simulink model "hw32a"  (R2017a)
settings: Solver=VariableStepAuto  StartTime=0.0  StopTime=10.0  RelTol=1e-3
undefined symbols (not defined in the file): sigbuilder_block
settings Model: Creator=Soutrik  LastModifiedBy=Soutrik

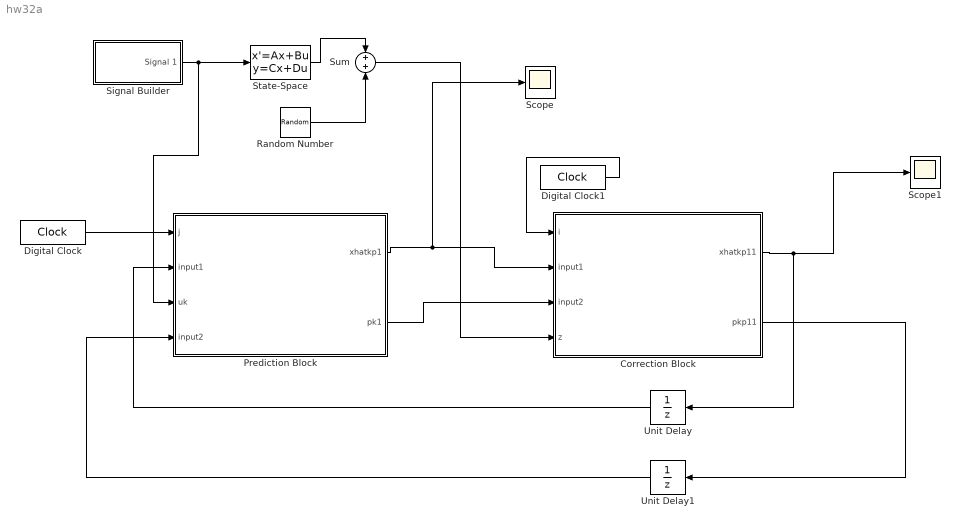
== system hw32a ==
  Correction Block : MATLAB Function  TreatAsAtomicUnit=on
  Digital Clock : DigitalClock  SampleTime=0.01
  Digital Clock1 : DigitalClock  SampleTime=0.01
  Prediction Block : MATLAB Function  TreatAsAtomicUnit=on
  Random Number : RandomNumber  Variance=[0.0001, 0.0000001, 0.00002, 0.00002]  SampleTime=0.01
  Scope : Scope
  Scope1 : Scope
  Signal Builder : Subsystem  Tag=STV Subsys  LoadFcn=sigbuilder_block('load');  StartFcn=sigbuilder_block('start');  StopFcn=sigbuilder_block('stop');  ClipboardFcn=sigbuilder_block('clipboard');  mask(Sigbuilder block){tuvar=[0:10]}
      mask help: Simulink:masks:SigbuilderBlock_MD
      mask init:
      | if ~strcmp(get_param(bdroot(gcbh),'SimulationStatus'),'stopped') tuvar = sigbuilder_block('maskInit'); end
      settings: CopyFcn=sigbuilder_block('copy');  DeleteFcn=sigbuilder_block('delete');  ModelCloseFcn=sigbuilder_block('modelClose');  PreSaveFcn=sigbuilder_block('preSave');  PauseFcn=sigbuilder_block('pause');  ContinueFcn=sigbuilder_block('continue');  NameChangeFcn=sigbuilder_block('namechange');  OpenFcn=sigbuilder_block('open',[300 184.875 550.5 400.125 ]);  CloseFcn=sigbuilder_block('close');
      mask Display: plot(0, 0, 100, 100,[2, 2, 32, 32, 2], [68, 8, 8, 68, 68],[32, 2], [38, 38], [32, 19, 2],[53, 60, 44], [32, 17, 17, 2],[16, 16, 31, 31]);txt = getActiveGroup(gcbh);text(2, 100, txt,'verticalAlignment', 'top');
  State-Space : StateSpace  A=|  B=|  C=|  D=[0;0;0;0];  X0=0
      A=|
      | [0 1.0000 0 0;
      | 0 -0.9965 0 -0.3000;
      | -0.3197 -0.5176 -0.0100 -0.7000;
      | 0 0 -0.0005 -0.9924];
      B=|
      | [ 0;
      | -0.0013;
      | 0.0001;
      | -0.0201];
      C=|
      | [0 0 0.9963 0.0862;
      | 0 0 -0.0001 0.0017;
      | 1.0000 0 0 0;
      | 0 1.0000 0 0];
  Sum : Sum  Inputs=2
  Unit Delay : UnitDelay  SampleTime=-1
  Unit Delay1 : UnitDelay  SampleTime=-1
  wires:
  Prediction Block/1(xhatkp1) -> Scope/1, Correction Block/2(input1)
  State-Space/1 -> Sum/1
  Random Number/1 -> Sum/2
  Signal Builder/1(Signal 1) -> Prediction Block/3(uk), State-Space/1
  Sum/1 -> Correction Block/4(z)
  Correction Block/1(xhatkp11) -> Scope1/1, Unit Delay/1
  Correction Block/2(pkp11) -> Unit Delay1/1
  Prediction Block/2(pk1) -> Correction Block/3(input2)
  Unit Delay/1 -> Prediction Block/2(input1)
  Unit Delay1/1 -> Prediction Block/4(input2)
  Digital Clock/1 -> Prediction Block/1(j)
  Digital Clock1/1 -> Correction Block/1(i)

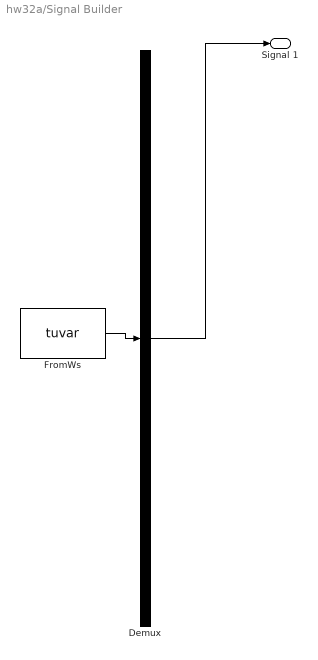
== system hw32a/Signal Builder ==
  Demux : Demux  Tag=STV Demux  Outputs=1
  FromWs : FromWorkspace  Tag=STV FromWs  VariableName=tuvar  SampleTime=0
      SigBuilderData=|
      | common.afterFinalStr = 'Extrapolate'
      | common.sampleTime = 0
      | dataSet.timeRange = [0 10]
      | dataSet.name = 'Group 1'
      | sbobj.Groups.Name = 'Group 1'
      | sbobj.Groups.Signals.Name = 'Signal 1'
      | sbobj.Groups.Signals.XData = [0 1.02 1.02 2.04 2.04 3.04 3.04 10]
      | sbobj.Groups.Signals.YData = [0 -0.002 50 50 -50 -50 0 0]
  Signal 1 : Outport  Tag=STV Outport
  wires:
  Demux/1 -> Signal 1/1
  FromWs/1 -> Demux/1

== matlab function hw32a/Correction Block ==
  data: i input; xhatkp11 output; input1 input; input2 input; pkp11 output; z input
function [xhatkp11, pkp11] = fcn(i,input1,input2,z)
xhatkp11=zeros(4,1);
pkp11=zeros(4);

if i<0.01
    
    xhatkp1=zeros(4,1);
    pkp1=eye(4);
else
    xhatkp1=input1;
    pkp1=input2;
end

c =[0 0 0.9963 0.0862;
0 0 -0.0001 0.0017;
1.0000 0 0 0;
0 1.0000 0 0];

h=c;
r=[0.0001, 0.0000001, 0.00002, 0.00002];
rk=diag(r);
ht=h';

kkp1=pkp1*ht*inv((h*pkp1*ht)+rk);
pkp11=(eye(4)-kkp1*h)*pkp1*(eye(4)-kkp1*h)'+kkp1*rk*(kkp1)';
xhatkp11=xhatkp1+kkp1*(z-h*xhatkp1);

end

== matlab function hw32a/Prediction Block ==
  data: j input; input1 input; xhatkp1 output; uk input; pk1 output; input2 input
function [xhatkp1,pk1] = fcn(j,input1,uk,input2)
xhatkp1=zeros(4,1);
pk1=zeros(4);

if j<0.01
    xhatk=zeros(4,1);
    pk=eye(4);
else
    xhatk=input1;
    pk=input2;
end

a = [0 1.0000 0 0;
0 -0.9965 0 -0.3000;
-0.3197 -0.5176 -0.0100 -0.7000;
0 0 -0.0005 -0.9924];
b =[ 0;
-0.0013;
0.0001;
-0.0201];

T=0.01;

ad=expm(a*T);
ainv=inv(a);
bd=(ainv).*(ad-eye(size(ad)))*b;
qk=eye(4);
pk=eye(4);



xhatkp1=ad*xhatk+bd*uk;
pk1=ad*pk*(ad)'+qk;
end
